simulink model "tc_4"  (Simulink 7.4)
settings: Solver=ode45  StartTime=0.0  StopTime=10.0  MaxStep=1/Fs  RelTol=1e-3
PreLoadFcn:
  | load  type_2_polynomials
  | Fs=1e3;
values from neighbouring files (symbols this model uses):
  Pfwd = [ +2.71443176145e-021, -1.25068871393e-017, +2.55744251786e-014, -3.31465196389e-011, +3.22028823036e-008, -2.32477968689e-005, +1.25934289740e-002, +5.40313308631e+000, +0.00000000000e+000 ]*1e-3    [Thermo_Couple_1.m]    (also in type_2_polynomials.mat = [2.71443176145e-24 -1.25068871393e-20 2.55744251786e-17 -3.3)
  Pinv_new = fit.coeff    [Thermo_Couple_1.m]    (also in type_2_polynomials.mat = [9.72907259059 -61.8281644488 165.304769177 -244.985065871 2)
undefined symbols (not defined in the file or in its folder): sigbuilder_block
libraries: simulink x2
settings Model: Creator=dbenson  LastModifiedBy=Dick
settings OptimizationCC: InitFltsAndDblsToZero=on
settings HardwareCC: ProdHWDeviceType=ASIC/FPGA->ASIC/FPGA  TargetEndianess=LittleEndian  TargetHWDeviceType=MATLAB Host  ProdEqTarget=off

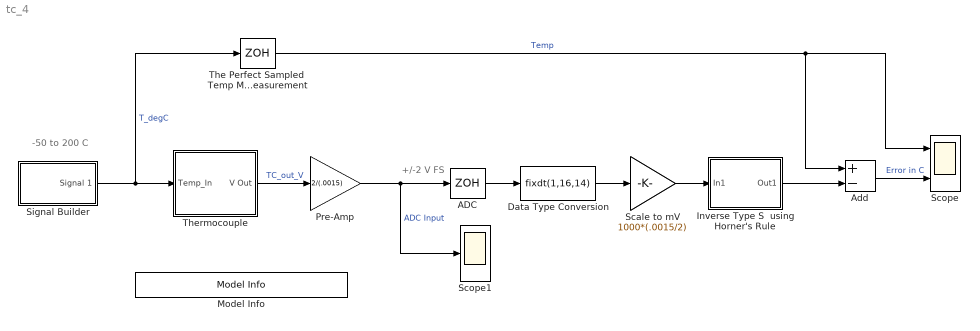
== system tc_4 ==
  note: +/-2 V FS
  note: -50 to 200 C
  ADC : ZeroOrderHold  SampleTime=1/Fs
  Add : Sum  Inputs=+-  OutDataType=sfix(16)  OutScaling=2^-10
  Data Type Conversion : DataTypeConversion  OutDataTypeMode=Specify via dialog  OutDataType=fixdt(1,16,14)  OutDataTypeStr=fixdt(1,16,14)  RndMeth=Nearest  SaturateOnIntegerOverflow=on
  "Inverse Type S  using Horner's Rule " : Subsystem  MinMaxOverflowLogging=MinMaxAndOverflow  mask{Pinv=Pinv_new, w=18, fl=9, wm=32}
      mask prompts: Pinv "Polynomial 9 th order"; w "number of bits in coefficients"; fl "number of bits in coef fraction"; wm "number of bits from mults"
      mask Display: disp('Horners Rule')
  Model Info : simulink/Model-Wide Utilities/Model Info  SystemSampleTime=-1  InitialBlockCM=None  BlockCM=None  Frame=on  DisplayStringWithTags=Copywrite 2005-2010 The MathWorks, Inc.  HorizontalTextAlignment=Center  LeftAlignmentValue=0.5  SourceBlockDiagram=tc_4  TagMaxNumber=20
  Pre-Amp : Gain  Gain=2/(.0015)  ParameterDataType=sfix(16)  ParameterScaling=2^0  OutDataType=sfix(16)  OutScaling=2^0
  Scale to mV : Gain  Gain=1000*(.0015/2)  ParameterDataTypeMode=Specify via dialog  ParameterDataType=fixdt(0,2,2)  ParamDataTypeStr=fixdt(0,2,2)  OutDataType=fixdt(1,16,15)  OutDataTypeStr=Inherit: Same as input
  Scope : Scope  NumInputPorts=2
      settings: TimeRange=10  YMin=-50~-0.05  YMax=200~0.03  MaxDataPoints=50000
  Scope1 : Scope
      settings: TimeRange=10  YMin=-2  YMax=2  MaxDataPoints=50000
  Signal Builder : Subsystem  Tag=STV Subsys  LoadFcn=sigbuilder_block('load',[20.25 252 448.5 274.5 ]);  StartFcn=sigbuilder_block('start');  StopFcn=sigbuilder_block('stop');  ClipboardFcn=sigbuilder_block('clipboard');  mask(Sigbuilder block){}
      mask help: Sigbuilder GUI
      mask init:
      | if ~strcmp(get_param(bdroot(gcbh),'SimulationStatus'),'stopped') tuvar = sigbuilder_block('maskInit'); end
      settings: CopyFcn=sigbuilder_block('copy');  DeleteFcn=sigbuilder_block('delete');  ModelCloseFcn=sigbuilder_block('modelClose');  PreSaveFcn=sigbuilder_block('preSave');  NameChangeFcn=sigbuilder_block('namechange');  OpenFcn=sigbuilder_block('open',[124.5 153 550.5 363.75 ]);  CloseFcn=sigbuilder_block('close');
      mask Display: plot(0,0,100,100,[10,10,40,40,10],[80,20,20,80,80],[40,10],[50,50], [40,27,10],[65,72,56],[40,25,25,10],[28,28,43,43]);
  The Perfect Sampled  Temp Measurement : ZeroOrderHold  SampleTime=1/Fs
  Thermocouple : Subsystem
  wires:
  Signal Builder/1(Signal 1) -> Thermocouple/1(Temp_In), The Perfect Sampled  Temp Measurement/1  "T_degC"
  Thermocouple/1(V Out) -> Pre-Amp/1  "TC_out_V"
  "Inverse Type S  using Horner's Rule "/1(Out1) -> Add/2
  Add/1 -> Scope/2  "Error in C"
  ADC/1 -> Data Type Conversion/1
  The Perfect Sampled  Temp Measurement/1 -> Add/1, Scope/1  "Temp"
  Pre-Amp/1 -> ADC/1, Scope1/1  "ADC Input"
  Scale to mV/1 -> "Inverse Type S  using Horner's Rule "/1(In1)
  Data Type Conversion/1 -> Scale to mV/1

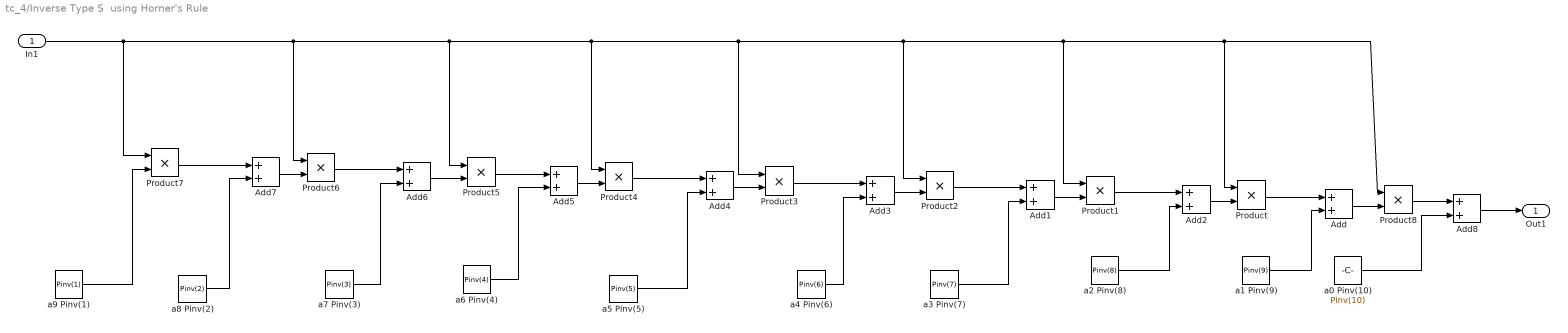
== system tc_4/Inverse Type S  using Horner's Rule  ==
  In1 : Inport
  Add{,1..7} (8 alike) : Sum  OutDataType=sfix(16)  OutScaling=2^-10
  Add8 : Sum  OutDataTypeMode=Specify via dialog  OutDataType=fixdt(1,wm,22)  OutDataTypeStr=fixdt(1,wm,22)
  Product : Product  OutDataTypeMode=Specify via dialog  OutDataType=fixdt(1,wm,25)  OutDataTypeStr=fixdt(1,wm,25)  RndMeth=Zero
  Product1 : Product  OutDataTypeMode=Specify via dialog  OutDataType=fixdt(1,wm,25)  OutDataTypeStr=fixdt(1,wm,25)  RndMeth=Zero
  Product2 : Product  OutDataTypeMode=Specify via dialog  OutDataType=fixdt(1,wm,24)  OutDataTypeStr=fixdt(1,wm,24)  RndMeth=Zero
  Product3 : Product  OutDataTypeMode=Specify via dialog  OutDataType=fixdt(1,wm,23)  OutDataTypeStr=fixdt(1,wm,23)  RndMeth=Zero
  Product4 : Product  OutDataTypeMode=Specify via dialog  OutDataType=fixdt(1,wm,23)  OutDataTypeStr=fixdt(1,wm,23)  RndMeth=Zero
  Product5 : Product  OutDataTypeMode=Specify via dialog  OutDataType=fixdt(1,wm,23)  OutDataTypeStr=fixdt(1,wm,23)  RndMeth=Zero
  Product6 : Product  OutDataTypeMode=Specify via dialog  OutDataType=fixdt(1,wm,24)  OutDataTypeStr=fixdt(1,wm,24)  RndMeth=Zero
  Product7 : Product  OutDataTypeMode=Specify via dialog  OutDataType=fixdt(1,wm,26)  OutDataTypeStr=fixdt(1,wm,26)  RndMeth=Zero
  Product8 : Product  OutDataTypeMode=Specify via dialog  OutDataType=fixdt(1,wm,22)  OutDataTypeStr=fixdt(1,wm,22)  RndMeth=Zero
  a0 Pinv(10) : Constant  Value=Pinv(10)  OutDataTypeMode=Specify via dialog  OutDataType=fixdt(1,w,fl)  ConRadixGroup=Best Precision: Vector-wise  OutDataTypeStr=fixdt(1,w,fl)  SampleTime=-1
  a1 Pinv(9) : Constant  Value=Pinv(9)  OutDataTypeMode=Specify via dialog  OutDataType=fixdt(1,w,fl)  ConRadixGroup=Best Precision: Vector-wise  OutDataTypeStr=fixdt(1,w,fl)  SampleTime=-1
  a2 Pinv(8) : Constant  Value=Pinv(8)  OutDataTypeMode=Specify via dialog  OutDataType=fixdt(1,w,fl)  ConRadixGroup=Best Precision: Vector-wise  OutDataTypeStr=fixdt(1,w,fl)  SampleTime=-1
  a3 Pinv(7) : Constant  Value=Pinv(7)  OutDataTypeMode=Specify via dialog  OutDataType=fixdt(1,w,fl)  ConRadixGroup=Best Precision: Vector-wise  OutDataTypeStr=fixdt(1,w,fl)  SampleTime=-1
  a4 Pinv(6) : Constant  Value=Pinv(6)  OutDataTypeMode=Specify via dialog  OutDataType=fixdt(1,w,fl)  ConRadixGroup=Best Precision: Vector-wise  OutDataTypeStr=fixdt(1,w,fl)  SampleTime=-1
  a5 Pinv(5) : Constant  Value=Pinv(5)  OutDataTypeMode=Specify via dialog  OutDataType=fixdt(1,w,fl)  ConRadixGroup=Best Precision: Vector-wise  OutDataTypeStr=fixdt(1,w,fl)  SampleTime=-1
  a6 Pinv(4) : Constant  Value=Pinv(4)  OutDataTypeMode=Specify via dialog  OutDataType=fixdt(1,w,fl)  ConRadixGroup=Best Precision: Vector-wise  OutDataTypeStr=fixdt(1,w,fl)  SampleTime=-1
  a7 Pinv(3) : Constant  Value=Pinv(3)  OutDataTypeMode=Specify via dialog  OutDataType=fixdt(1,w,fl)  ConRadixGroup=Best Precision: Vector-wise  OutDataTypeStr=fixdt(1,w,fl)  SampleTime=-1
  a8 Pinv(2) : Constant  Value=Pinv(2)  OutDataTypeMode=Specify via dialog  OutDataType=fixdt(1,w,fl)  ConRadixGroup=Best Precision: Vector-wise  OutDataTypeStr=fixdt(1,w,fl)  SampleTime=-1
  a9 Pinv(1) : Constant  Value=Pinv(1)  OutDataTypeMode=Specify via dialog  OutDataType=fixdt(1,w,fl)  ConRadixGroup=Best Precision: Vector-wise  OutDataTypeStr=fixdt(1,w,fl)  SampleTime=-1
  Out1 : Outport
  wires:
  a0 Pinv(10)/1 -> Add8/2
  Add8/1 -> Out1/1
  Product8/1 -> Add8/1
  Add/1 -> Product8/2
  a9 Pinv(1)/1 -> Product7/2
  Product7/1 -> Add7/1
  a8 Pinv(2)/1 -> Add7/2
  Add7/1 -> Product6/2
  Product6/1 -> Add6/1
  a7 Pinv(3)/1 -> Add6/2
  Add6/1 -> Product5/2
  a6 Pinv(4)/1 -> Add5/2
  Product5/1 -> Add5/1
  Add5/1 -> Product4/2
  Product4/1 -> Add4/1
  a5 Pinv(5)/1 -> Add4/2
  Add4/1 -> Product3/2
  Product3/1 -> Add3/1
  a4 Pinv(6)/1 -> Add3/2
  Add3/1 -> Product2/2
  Product2/1 -> Add1/1
  a3 Pinv(7)/1 -> Add1/2
  Add1/1 -> Product1/2
  Product1/1 -> Add2/1
  Add2/1 -> Product/2
  a2 Pinv(8)/1 -> Add2/2
  In1/1 -> Product7/1, Product6/1, Product5/1, Product4/1, Product3/1, Product2/1, Product8/1, Product/1, Product1/1
  Product/1 -> Add/1
  a1 Pinv(9)/1 -> Add/2

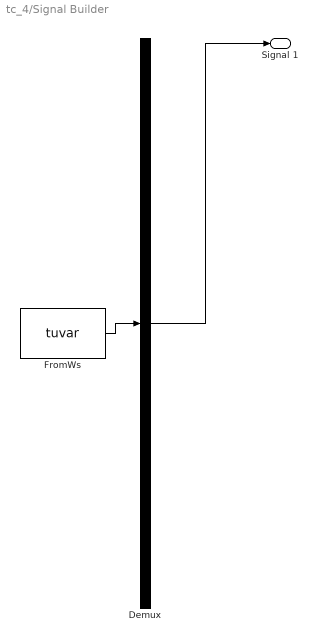
== system tc_4/Signal Builder ==
  Demux : Demux  Tag=STV Demux  Outputs=1
  FromWs : FromWorkspace  Tag=STV FromWs  VariableName=tuvar  SampleTime=0  SigBuilderData=DataTag0  VnvData=DataTag1
      SigBuilderData=|
      | common.afterFinalStr = 'Extrapolate'
      | common.sampleTime = 0
      | dataSet.timeRange = [0 10]
      | dataSet.name = 'Group 1'
      | sbobj.Groups.Name = 'Group 1'
      | sbobj.Groups.Signals.Name = 'Signal 1'
      | sbobj.Groups.Signals.XData = [0 1.7 5 8.1 10]
      | sbobj.Groups.Signals.YData = [-50 -50 200 -50 -50]
  Signal 1 : Outport  Tag=STV Outport  OutDataType=sfix(16)  OutScaling=2^0
  wires:
  Demux/1 -> Signal 1/1
  FromWs/1 -> Demux/1

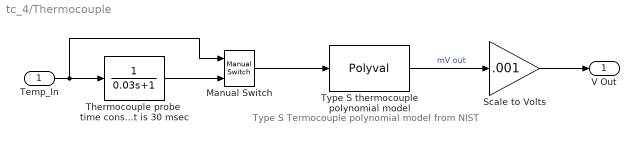
== system tc_4/Thermocouple ==
  note: Type S Termocouple
      | polynomial model
      | from NIST
  Temp_In : Inport
  Manual Switch : simulink/Signal Routing/Manual Switch  SystemSampleTime=-1  sw=1  action=0  varsize=off
  Scale to Volts : Gain  Gain=.001  ParameterDataType=sfix(16)  ParameterScaling=2^0  OutDataType=sfix(16)  OutScaling=2^0
  Thermocouple probe  time constant is 30 msec : TransferFcn  Denominator=[0.03 1]
  Type S thermocouple polynomial model : Polyval  Coefs=Pfwd
      settings: AttributesFormatString=%<Description>
  V Out : Outport
  wires:
  Temp_In/1 -> Thermocouple probe  time constant is 30 msec/1, Manual Switch/1
  Type S thermocouple polynomial model/1 -> Scale to Volts/1  "mV out"
  Thermocouple probe  time constant is 30 msec/1 -> Manual Switch/2
  Manual Switch/1 -> Type S thermocouple polynomial model/1
  Scale to Volts/1 -> V Out/1
